simulink model "final_2"  (R2020a)
settings: Solver=VariableStepAuto  StartTime=0.0  StopTime=4  RelTol=1e-3
undefined symbols (not defined in the file): fdesignblkfcn, gcbh
libraries: dspvision x5, dspfdesign x2, audiosources x1, dspsnks4 x1, dsparch4 x1, dspsrcs4 x1
settings Model: Creator=Karan  LastModifiedBy=Karan

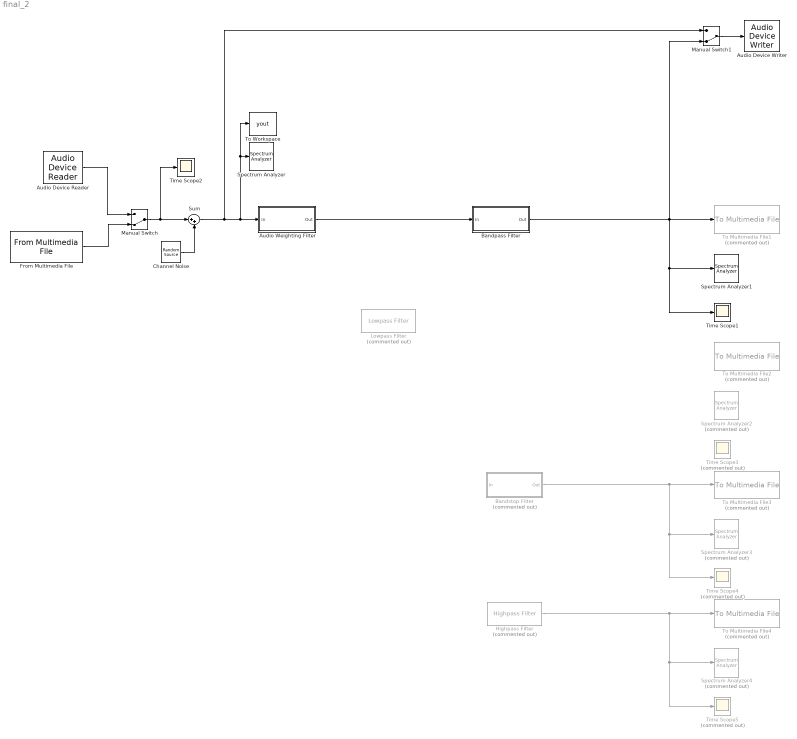
== system final_2 ==
  Audio Device Reader : audiosources/Audio Device Reader  Driver=DirectSound  Device=Default  SampleRate=44100  NumChannels=1  SamplesPerFrame=1024  BitDepth=16-bit integer  NumBuffers=10  DefaultInputChannelMapping=on  InputChannelMapping=1:2  OutputNumOverrunSamples=off  OutputDataType=double  DriverIdx=1  DeviceWarnFlag=''
      settings: SourceProductBaseCode=AU
  Audio Device Writer : dspsnks4/Audio Device Writer  Driver=DirectSound  Device=Default  InheritSampleRate=off  SampleRate=8000  BitDepth=16-bit integer  BufferSize=4096  NumBuffers=10  DefaultOutputChannelMapping=on  OutputChannelMapping=1:2  OutputNumUnderrunSamples=off  DriverIdx=1  DeviceWarnFlag=''
  Audio Weighting Filter : Subsystem  DialogController=fdesignblkfcn  InitFcn=fdesignblkfcn(gcbh, {'InitFcn'});  mask(Audio Weighting Filter){}
      mask help: Design an audio weighting filter
      settings: CopyFcn=fdesignblkfcn(gcbh, {'CopyFcn'});
      mask Help: helpview(mapfilelocation('dsp'), 'dspaudioweightingfilter');
      mask Display: disp('Audio Weighting')
  Bandpass Filter : Subsystem  DialogController=fdesignblkfcn  InitFcn=fdesignblkfcn(gcbh, {'InitFcn'});  mask(Bandpass Filter){}
      mask help: Design a bandpass filter
      settings: CopyFcn=fdesignblkfcn(gcbh, {'CopyFcn'});
      mask Help: helpview(mapfilelocation('dsp'), 'dspbandpassfilter');
      mask Display: disp('Bandpass');
  Bandstop Filter : Subsystem  Commented=on  DialogController=fdesignblkfcn  InitFcn=fdesignblkfcn(gcbh, {'InitFcn'});  mask(Bandstop Filter){}
      mask help: Design a bandstop filter
      settings: CopyFcn=fdesignblkfcn(gcbh, {'CopyFcn'});
      mask Help: helpview(mapfilelocation('dsp'), 'dspbandstopfilter');
      mask Display: disp('Bandstop');
  Channel Noise : dspsrcs4/Random Source  SrcType=Gaussian  NormMethod=Ziggurat  CltLength=12  MinVal=0  MaxVal=1  MeanVal=0  VarVal=0.0005  RepMode=Not repeatable  rawSeed=1  IsInherit=on  SampMode=Discrete  SampTime=1/8000  SampFrame=1024  DataType=Double  OutComplex=Real  OutputFrames=off
  From Multimedia File : dspvision/From Multimedia File  inputFilename=C:\Users\Karan\Downloads\babble_5dB\5dB\sp02_babble_sn5.wav  readRange=[1 Inf]  loop=on  numPlays=inf  outputStreams=Audio only  videoDataType=single  audioDataType=double  inheritSampleTime=on  userDefinedSampleTime=1/44100  noAudioOutput=off  isIntensityVideo=off  fourcc=RGB  colorVideoFormat=Separate color signals  outputEOF=off  dataOrg=Column-major  audioFrameSize=1024  computeAudioFrameSize=off  outSamplingMode=Sample based
  Highpass Filter : dspfdesign/Highpass Filter  Commented=on  FilterType=FIR  DesignForMinimumOrder=on  FilterOrder=50  StopbandFrequency=8e3  PassbandFrequency=12e3  StopbandAttenuation=80  PassbandRipple=0.1  InheritSampleRate=off  SampleRate=44100  SimulateUsing=Interpreted execution  roundingMode=Floor  coeffsDataTypeStr=fixdt(1,16)
  Lowpass Filter : dspfdesign/Lowpass Filter  Commented=on  FilterType=FIR  DesignForMinimumOrder=on  FilterOrder=50  PassbandFrequency=3400  StopbandFrequency=6000  PassbandRipple=0.1  StopbandAttenuation=80  InheritSampleRate=off  SampleRate=44100  SimulateUsing=Interpreted execution  roundingMode=Floor  coeffsDataTypeStr=fixdt(1,16)
  Manual Switch : ManualSwitch  CurrentSetting=0
  Manual Switch1 : ManualSwitch  CurrentSetting=0
  Spectrum Analyzer : SpectrumAnalyzer
  Spectrum Analyzer1 : SpectrumAnalyzer
  Spectrum Analyzer2 : SpectrumAnalyzer  Commented=on
  Spectrum Analyzer3 : SpectrumAnalyzer  Commented=on
  Spectrum Analyzer4 : SpectrumAnalyzer  Commented=on
  Sum : Sum  Inputs=|++
  Time Scope1 : Scope
  Time Scope2 : Scope
  Time Scope3 : Scope  Commented=on
  Time Scope4 : Scope  Commented=on
  Time Scope5 : Scope  Commented=on
  To Multimedia File{1..4} (4 alike) : dspvision/To Multimedia File  Commented=on  outputFilename=D:\projects_on_github\tri-8_project\Matlab\LowPassOutput.wav  streamSelection=Audio only  videoCompressor=None (uncompressed)  audioCompressor=None (uncompressed)  imagePorts=Separate color signals  fileType=WAV  audioDatatype=16-bit integer  fourcc=RGB  videoQuality=75  mj2000CompFactor=10
  To Workspace : ToWorkspace  VariableName=yout  SampleTime=-1
      settings: Save2DSignal=2-D array (concatenate along first dimension)
  wires:
  From Multimedia File/1 -> Manual Switch/2
  Audio Device Reader/1 -> Manual Switch/1
  Channel Noise/1 -> Sum/2
  Manual Switch/1 -> Time Scope2/1, Sum/1
  Manual Switch1/1 -> Audio Device Writer/1
  ? -> To Multimedia File2/1, Spectrum Analyzer2/1, Time Scope3/1
  Bandstop Filter/1(Out) -> Spectrum Analyzer3/1, Time Scope4/1, To Multimedia File3/1
  Highpass Filter/1 -> Spectrum Analyzer4/1, Time Scope5/1, To Multimedia File4/1
  Sum/1 -> Manual Switch1/1, Audio Weighting Filter/1(In), To Workspace/1, Spectrum Analyzer/1
  Audio Weighting Filter/1(Out) -> Bandpass Filter/1(In)
  Bandpass Filter/1(Out) -> Spectrum Analyzer1/1, Time Scope1/1, Manual Switch1/2, To Multimedia File1/1

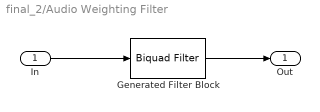
== system final_2/Audio Weighting Filter ==
  In : Inport
  Generated Filter Block : dsparch4/Biquad Filter  Tag=BlockMethodSubSystem  FilterSource=Dialog parameters  CoeffSource=Specify via dialog  FilterObject=BQF  IIRFiltStruct=Direct form II  BiQuadCoeffs=[1.24652229185234664 0 -1.24652229185234664 1 0.103818049793350742 -0.360417438157730807;0.0471337743318483784 0 -0.0471337743318483784 1 -0.26438243082112467 -0.601403461744298373;1 -2 1 1 -1.96790281198134798 0.968160369351024119]  ScaleValues=[0.535764719033171022;1;1;20.0337390876515293]  IC=0  ICnum=0  ICden=0  a0Flag=Warning  optimizeScaleValues=off  ScaleValueMode=Specify via input port (g)  InputProcessing=Columns as channels (frame based)  roundingMode=Floor  overflowMode=off  scaleValueFracLength=14  denProdOutputFracLength=30  denAccumFracLength=30  secondMemoryFracLength=15
  Out : Outport  VectorParamsAs1DForOutWhenUnconnected=off
  wires:
  In/1 -> Generated Filter Block/1
  Generated Filter Block/1 -> Out/1

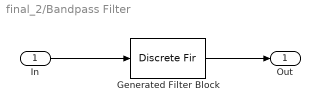
== system final_2/Bandpass Filter ==
  In : Inport
  Generated Filter Block : DiscreteFir  Tag=BlockMethodSubSystem  Coefficients=[-0.0186837625677451769 -0.0116138989269169261 0.00822962473465216338 -0.00547573568862816124 0.00445155071872786485 0.000240892027910798168 0.00150359114776866393 0.00629624147279927819 -0.000551636308459416309 0.0111288984122155966 -3.93772626611204463e-05 0.0122887238045168677 0.00435040075459419869 0.00874210927395818564 0.0114609684872962227 0.00239865356772412178 0.0172370012745991855 -0.0025214680584704505 0.0166311235199305026 -0.00223985910241264463 0.00698139858518614237 0.00335800468265919777 -0.00928741030410205545 0.0092510072039275696 -0.0249864738696606511 0.0073697380148752302 -0.0316555747024144032 -0.00837534997493204897 -0.0252151968182521141 -0.0372099357422484567 -0.00997459792217696845 -0.0689617954692126472 0.001172905801351945 -0.0865243989860606105 -0.00935839758786052855 -0.0700538484330945205 -0.0621945355365921548 0.0107539365195831321 -0.226805525371005567 0.567446591558775415 0.567446591558775415 -0.226805525371005567 0.0107539365195831321 -0.0621945355365921548 -0.0700538484330945205 -0.00935839758786052855 -0.0865243989860606105 0.001172905801351945 -0.0689617954692126472 -0.00997459792217696845 -0.0372099357422484567 -0.0252151968182521141 -0.00837534997493204897 -0.0316555747024144032 0.0073697380148752302 -0.0249864738696606511 0.0092510072039275696 -0.00928741030410205545 0.00335800468265919777 0.00698139858518614237 -0.00223985910241264463 0.0166311235199305026 -0.0025214680584704505 0.0172370012745991855 0.00239865356772412178 0.0114609684872962227 0.00874210927395818564 0.00435040075459419869 0.0122887238045168677 -3.93772626611204463e-05 0.0111288984122155966 -0.000551636308459416309 0.00629624147279927819 0.00150359114776866393 0.000240892027910798168 0.00445155071872786485 -0.00547573568862816124 0.00822962473465216338 -0.0116138989269169261 -0.0186837625677451769]  InputProcessing=Columns as channels (frame based)
  Out : Outport  VectorParamsAs1DForOutWhenUnconnected=off
  wires:
  In/1 -> Generated Filter Block/1
  Generated Filter Block/1 -> Out/1

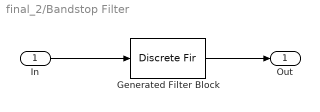
== system final_2/Bandstop Filter ==
  In : Inport
  Generated Filter Block : DiscreteFir  Tag=BlockMethodSubSystem  Coefficients=[-0.00049984690227566171 9.5100318056220678e-05 -0.018778888889125381 0.00020561736622238936 0.0019605411941885044 0.00023848464356614288 0.011427768692370117 0.00024928020776728103 -0.026344143468356181 0.00022323473160311075 0.033802321854574921 0.00024455404571586617 -0.019823660150560137 0.00024377045334422507 -0.019896328302992174 0.00022786848806407702 0.082714162332194516 0.00025656261277749384 -0.15101859373266049 0.00022072984516862497 0.20526035643478094 0.0002476136866061962 0.77489283142488197 0.0002476136866061962 0.20526035643478094 0.00022072984516862497 -0.15101859373266049 0.00025656261277749384 0.082714162332194516 0.00022786848806407702 -0.019896328302992174 0.00024377045334422507 -0.019823660150560137 0.00024455404571586617 0.033802321854574921 0.00022323473160311075 -0.026344143468356181 0.00024928020776728103 0.011427768692370117 0.00023848464356614288 0.0019605411941885044 0.00020561736622238936 -0.018778888889125381 9.5100318056220678e-05 -0.00049984690227566171]  InputProcessing=Columns as channels (frame based)
  Out : Outport  VectorParamsAs1DForOutWhenUnconnected=off
  wires:
  Generated Filter Block/1 -> Out/1
  In/1 -> Generated Filter Block/1
